simulink model "ObtenerDatosSensores"  (R2020b)
settings: Solver=VariableStepAuto  StartTime=0.0  StopTime=10.0  RelTol=1e-3
settings Model: Creator=sergi  LastModifiedBy=sergi

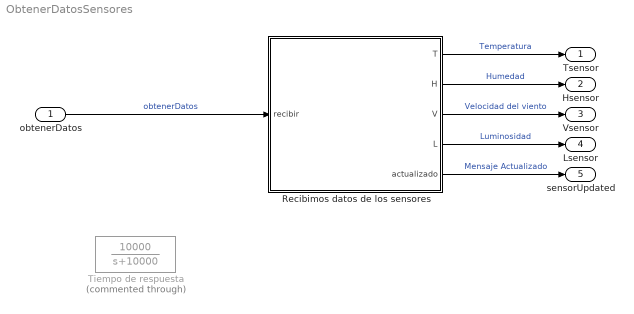
== system ObtenerDatosSensores ==
  "obtenerDatos " : Inport  OutMin=0  OutMax=72  OutDataTypeStr=double  PortDimensions=1
  Recibimos datos de los sensores : MATLAB Function  TreatAsAtomicUnit=on
  Tiempo de respuesta : TransferFcn  Commented=through  Numerator=[10000]  Denominator=[1 10000]
  Tsensor : Outport  SignalName=Tsensor  OutMin=0  OutMax=35  OutDataTypeStr=double  PortDimensions=1
      settings: MustResolveToSignalObject=on
  Hsensor : Outport  Port=2  SignalName=Hsensor  OutMin=0  OutMax=1  OutDataTypeStr=double  PortDimensions=1
      settings: MustResolveToSignalObject=on
  Vsensor : Outport  Port=3  SignalName=Vsensor  OutMin=0  OutMax=1  OutDataTypeStr=double  PortDimensions=1
      settings: MustResolveToSignalObject=on
  Lsensor : Outport  Port=4  SignalName=Lsensor  OutMin=0  OutMax=1  OutDataTypeStr=double  PortDimensions=1
      settings: MustResolveToSignalObject=on
  sensorUpdated : Outport  Port=5  SignalName=sensorUpdated  OutMin=0  OutMax=1  PortDimensions=1
      settings: MustResolveToSignalObject=on
  wires:
  Recibimos datos de los sensores/2(H) -> Hsensor/1  "Humedad"
  Recibimos datos de los sensores/1(T) -> Tsensor/1  "Temperatura"
  "obtenerDatos "/1 -> Recibimos datos de los sensores/1(recibir)  "obtenerDatos"
  Recibimos datos de los sensores/5(actualizado) -> sensorUpdated/1  "Mensaje Actualizado"
  Recibimos datos de los sensores/3(V) -> Vsensor/1  "Velocidad del viento"
  Recibimos datos de los sensores/4(L) -> Lsensor/1  "Luminosidad"

== matlab function ObtenerDatosSensores/Recibimos datos de los sensores ==
  settings: updateMethod=DISCRETE
  data: recibir input; T output; H output; V output; L output; actualizado output
function [T,H,V,L,actualizado] = RecibirDatosSensores(recibir)

persistent x0

no_error = 1;

if no_error && recibir
    
    if isempty(x0)
        x0=1651255;
    end
    
    m=2^31;
    x0=rem(314159269*x0+453806245,m);
    uniforme=x0/m;
    T = 0 + uniforme * 35;  % Temperatura
    
    m=2^31;
    x0=rem(314159269*x0+453806245,m);
    uniforme=x0/m;
    H = uniforme;           % Humedad
    
    m=2^31;
    x0=rem(314159269*x0+453806245,m);
    uniforme=x0/m;
    V = uniforme*1.6;       % Viento
    
    m=2^31;
    x0=rem(314159269*x0+453806245,m);
    uniforme=x0/m;
    L = uniforme;           % Luminosidad
    
    actualizado = 1;
else
    T = [0];
    H = [0];
    V = [0];
    L = [0];
    actualizado = 0;
end

end
